simulink model "Aprox_PWM_Motor_Driver_Circu"  (R2014b)
settings: Solver=ode45  StartTime=0.0  StopTime=.3  MaxStep=.0001  RelTol=1e-3
values from neighbouring files (symbols this model uses):
  Vcc = 24    [motorParams.m]

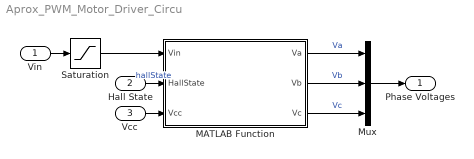
== system Aprox_PWM_Motor_Driver_Circu ==
  Vin : Inport  OutDataTypeStr=double  PortDimensions=1  SampleTime=0
  Hall State : Inport  Port=2  OutDataTypeStr=double  PortDimensions=[1 3]  SampleTime=0
  Vcc : Inport  Port=3  OutDataTypeStr=double  PortDimensions=1  SampleTime=[0,0]
  MATLAB Function : MATLAB Function  TreatAsAtomicUnit=on
  Mux : Mux  Inputs=3
  Saturation : Saturate  UpperLimit=Vcc  LowerLimit=-Vcc
  Phase Voltages : Outport  OutDataTypeStr=double  PortDimensions=3  SampleTime=0
  wires:
  Saturation/1 -> MATLAB Function/1(Vin)
  Hall State/1 -> MATLAB Function/2(HallState)  "hallState"
  Vin/1 -> Saturation/1
  Vcc/1 -> MATLAB Function/3(Vcc)
  MATLAB Function/2(Vb) -> Mux/2  "Vb"
  MATLAB Function/1(Va) -> Mux/1  "Va"
  MATLAB Function/3(Vc) -> Mux/3  "Vc"
  Mux/1 -> Phase Voltages/1

== matlab function Aprox_PWM_Motor_Driver_Circu/MATLAB Function ==
function [Va, Vb, Vc] = halfBridge(Vin, HallState, Vcc)

    if isequal(HallState, [1, 0, 0])
        Va = Vin/2;
        Vb = -Vin/2;
        Vc = 0;
    elseif isequal(HallState, [1, 1, 0])
        Va = Vin/2;
        Vb = 0;
        Vc = -Vin/2;
    elseif isequal(HallState, [0, 1, 0])
        Va = 0;
        Vb = Vin/2;
        Vc = -Vin/2;
    elseif isequal(HallState, [0, 1, 1])
        Va = -Vin/2;
        Vb = Vin/2;
        Vc = 0;
    elseif isequal(HallState, [0, 0, 1])
        Va = -Vin/2;
        Vb = 0;
        Vc = Vin/2;
    elseif  isequal(HallState, [1, 0, 1])
        Va = 0;
        Vb = -Vin/2;
        Vc = Vin/2;
    else 
        Va = 0;
        Vb = 0;
        Vc = 0;
    end
end
